simulink model "pid0510"  (R2023a)
settings: Solver=VariableStepAuto  StartTime=0.0  StopTime=3  FixedStep=10^-3  RelTol=1e-3
undefined symbols (not defined in the file or in its folder): kd, ki, kp, T
settings Model: Creator=a2270170  LastModifiedBy=a2270170

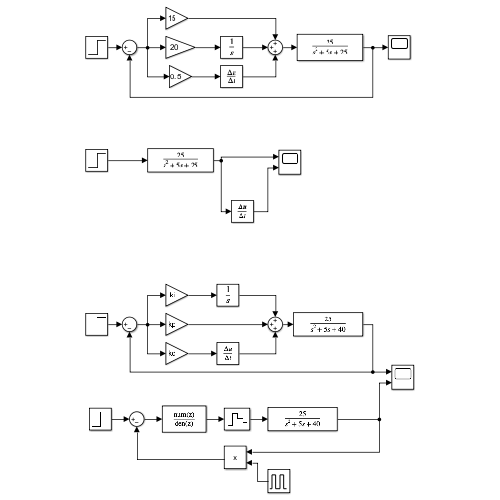
[thumbnail: Simulink's stored preview of the top-level diagram]
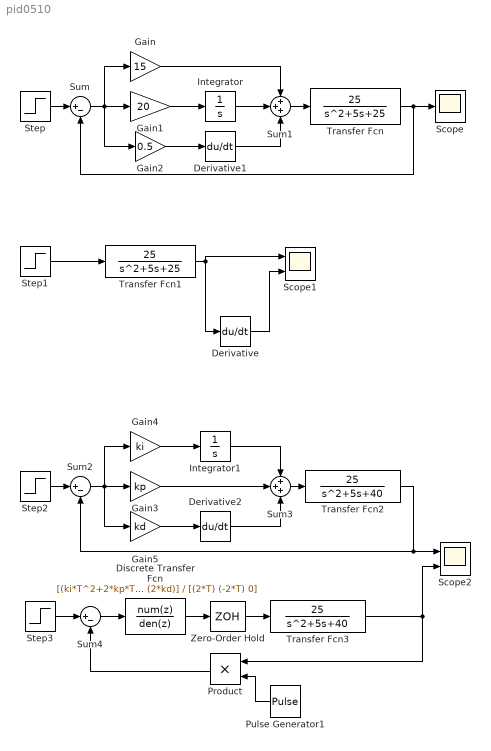
== system pid0510 ==
  Derivative : Derivative
  Derivative1 : Derivative
  Derivative2 : Derivative
  Discrete Transfer Fcn : DiscreteTransferFcn  Numerator=[(ki*T^2+2*kp*T+2*kd) (ki*T^2-2*kp*T-4*kd) (2*kd)]  Denominator=[(2*T) (-2*T) 0]  SampleTime=T
  Gain : Gain  Gain=15
  Gain1 : Gain  Gain=20
  Gain2 : Gain  Gain=0.5
  Gain3 : Gain  Gain=kp
  Gain4 : Gain  Gain=ki
  Gain5 : Gain  Gain=kd
  Integrator : Integrator
  Integrator1 : Integrator
  Product : Product
  Pulse Generator1 : DiscretePulseGenerator  PulseType=Time based  Period=T  PulseWidth=0.1
  Scope : Scope
  Scope1 : Scope  NumInputPorts=2
  Scope2 : Scope  NumInputPorts=2
  Step{,1..3} (4 alike) : Step  SampleTime=0
  Sum : Sum  Inputs=|+-
  Sum1 : Sum  Inputs=+++
  Sum2 : Sum  Inputs=|+-
  Sum3 : Sum  Inputs=+++
  Sum4 : Sum  Inputs=|+-
  Transfer Fcn : TransferFcn  Numerator=[25]  Denominator=[1 5 25]
  Transfer Fcn1 : TransferFcn  Numerator=[25]  Denominator=[1 5 25]
  Transfer Fcn2 : TransferFcn  Numerator=[25]  Denominator=[1 5 40]
  Transfer Fcn3 : TransferFcn  Numerator=[25]  Denominator=[1 5 40]
  Zero-Order Hold : ZeroOrderHold  SampleTime=T
  wires:
  Transfer Fcn1/1 -> Derivative/1, Scope1/1
  Step1/1 -> Transfer Fcn1/1
  Derivative/1 -> Scope1/2
  Sum/1 -> Gain2/1, Gain1/1, Gain/1
  Step/1 -> Sum/1
  Integrator/1 -> Sum1/2
  Gain1/1 -> Integrator/1
  Gain2/1 -> Derivative1/1
  Derivative1/1 -> Sum1/3
  Gain/1 -> Sum1/1
  Sum1/1 -> Transfer Fcn/1
  Transfer Fcn/1 -> Sum/2, Scope/1
  Gain4/1 -> Integrator1/1
  Step2/1 -> Sum2/1
  Transfer Fcn2/1 -> Sum2/2, Scope2/1
  Gain3/1 -> Sum3/2
  Integrator1/1 -> Sum3/1
  Sum2/1 -> Gain4/1, Gain3/1, Gain5/1
  Derivative2/1 -> Sum3/3
  Gain5/1 -> Derivative2/1
  Sum3/1 -> Transfer Fcn2/1
  Step3/1 -> Sum4/1
  Sum4/1 -> Discrete Transfer Fcn/1
  Discrete Transfer Fcn/1 -> Zero-Order Hold/1
  Zero-Order Hold/1 -> Transfer Fcn3/1
  Transfer Fcn3/1 -> Scope2/2, Product/1
  Pulse Generator1/1 -> Product/2
  Product/1 -> Sum4/2
